simulink model "sfunctionbuilder"  (R2018b)
settings: Solver=VariableStepAuto  StartTime=0.0  StopTime=10.0  RelTol=1e-3
settings Model: Creator=student  LastModifiedBy=student

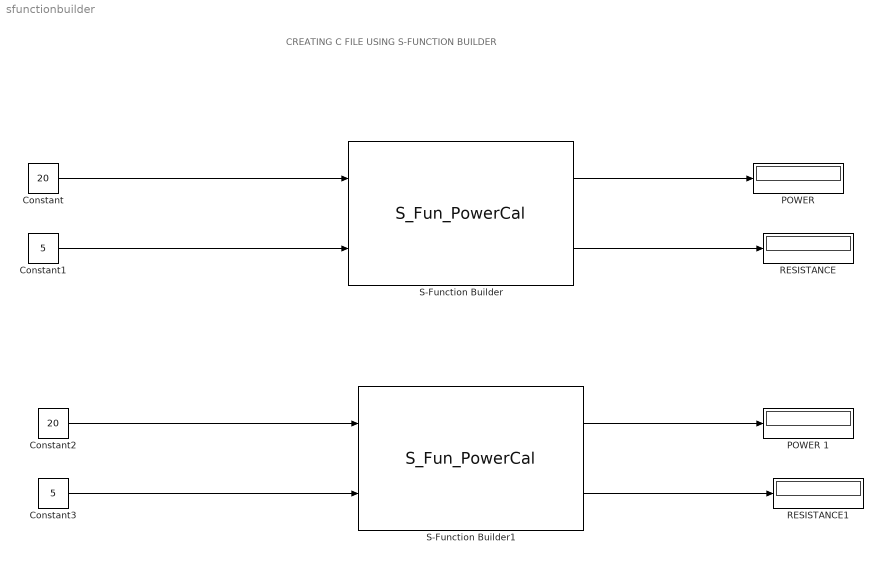
== system sfunctionbuilder ==
  note: CREATING C FILE USING S-FUNCTION BUILDER
  Constant : Constant  Value=20
  Constant1 : Constant  Value=5
  Constant2 : Constant  Value=20
  Constant3 : Constant  Value=5
  "POWER " : Display
  POWER 1 : Display
  RESISTANCE : Display
  RESISTANCE1 : Display
  S-Function Builder : S-Function  InitFcn=try, set_param(gcb,'FunctionName','S_Fun_PowerCal'), end  FunctionName=S_Fun_PowerCal  SFunctionModules=S_Fun_PowerCal_wrapper  SFunctionDeploymentMode=off  EnableBusSupport=off  mask(S-Function Builder){}
      mask help: Simulink:masks:SFunctionBuilder_MD
      mask init:
      | val = [[.9  0.75 0.75 1 1 .9 .9 1]',[1 1 0.75 0.75 .9 .9 1 .9]'];try , sys = get_param(gcb,'SfunBuilderFcnName');if isempty(sys), sys = get_param(gcb,'FunctionName'); end,catch, sys = get_param(gcb,'FunctionName'); end
      settings: CopyFcn=set_param(gcbh,'LinkStatus','none')  PreSaveFcn=try, set_param(gcb,'FunctionName','S_Fun_PowerCal'), end  OpenFcn=sfunctionwizard(gcbh)
      mask Display: plot(val(:,1),val(:,2)),disp(sys), port_label('input',1,'Voltage'), port_label('input',2,'Current'), port_label('output',1,'Power'), port_label('output',2,'Resistance')
  S-Function Builder1 : S-Function  InitFcn=try, set_param(gcb,'FunctionName','S_Fun_PowerCal'), end  FunctionName=S_Fun_PowerCal  SFunctionModules=S_Fun_PowerCal_wrapper  SFunctionDeploymentMode=off  EnableBusSupport=off  mask(S-Function Builder){}
      mask help: Simulink:masks:SFunctionBuilder_MD
      mask init: same as sfunctionbuilder/S-Function Builder
      settings: CopyFcn=set_param(gcbh,'LinkStatus','none')  PreSaveFcn=try, set_param(gcb,'FunctionName','S_Fun_PowerCal'), end  OpenFcn=sfunctionwizard(gcbh)
      mask Display:
      | plot(val(:,1),val(:,2))
      | disp(sys)
      | port_label('input',1,'Voltage')
      | port_label('input',2,'Current')
      | port_label('output',1,'Power')
      | port_label('output',2,'Resistance')
      | image('Penguins.jpg')
  wires:
  S-Function Builder/1 -> "POWER "/1
  S-Function Builder/2 -> RESISTANCE/1
  Constant/1 -> S-Function Builder/1
  Constant1/1 -> S-Function Builder/2
  Constant3/1 -> S-Function Builder1/2
  Constant2/1 -> S-Function Builder1/1
  S-Function Builder1/1 -> POWER 1/1
  S-Function Builder1/2 -> RESISTANCE1/1
